simulink model "coremodel"  (R2026a)
settings: Solver=ode23t  StopTime=12  MaxStep=1e-4  RelTol=1e-4
values from neighbouring files (symbols this model uses):
  Bshaft = 2000    [init.m]    (also in isolator_config_demo.m)
  TorqueFullScaleNm = 10000    [init.m]    (also in isolator_config_demo.m)
  Ts = 0.001    [init.m]    (also in isolator_config_demo.m)
libraries: fl_lib x16, nesl_utility x10, ee_lib x1
settings Model: Creator=saranya  LastModifiedBy=saranya

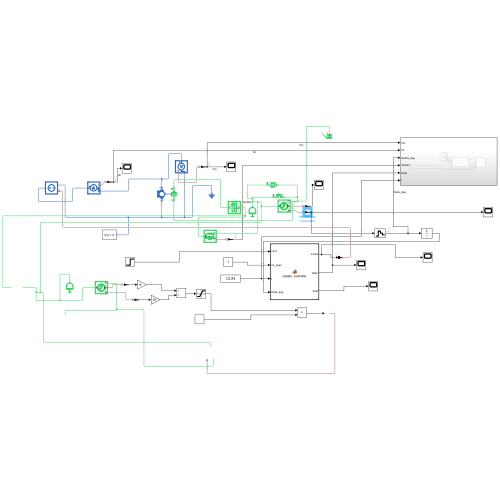
[thumbnail: Simulink's stored preview of the top-level diagram]
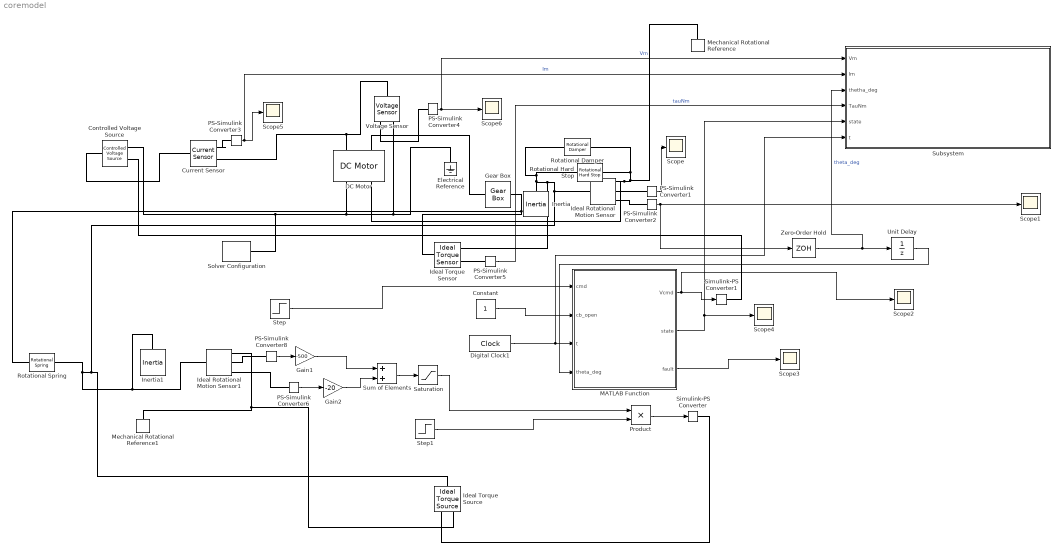
== system coremodel ==
  Constant : Constant
  Controlled Voltage Source : fl_lib/Electrical/Electrical Sources/Controlled Voltage Source
  Current Sensor : fl_lib/Electrical/Electrical Sensors/Current Sensor
  DC Motor : ee_lib/Electromechanical/Brushed Motors/DC Motor  field_option=ee.enum.field_option.pm  Rf=100 Ohm  Lf=1 H  Laf=0.15 H  If0=0 A  parameterization=ee.enum.dcparam_option.circuit_param  Ra=5 Ohm  La=0.05 H  emf_or_torque=ee.enum.emf_or_torque.ki  Kv=0.072e-3 V/rpm  Ki=0.5 N*m/A  T_stall=0.24e-3 N*m  w_max=19100 rpm  w_rated=15000 rpm  P_rated=0.08 W  V_rated=1.5 V  lam_param=ee.enum.lam_param.damping  i_noload=0 A  V_i_noload=1.5 V  J=0.002 cm^2*g  lam=0.001 N*m*s/rad  speed0=0 rpm  alpha=3.93e-3 1/K  Tmeas=25 degC  thermal_mass=100 J/K  initial_temperature=25 degC
  Digital Clock1 : DigitalClock
  Electrical Reference : fl_lib/Electrical/Electrical Elements/Electrical Reference
  Gain1 : Gain  Gain=-500
  Gain2 : Gain  Gain=-20
  Gear Box : fl_lib/Mechanical/Mechanisms/Gear Box  ratio=600  t_in_specify=off  t_in_priority=None  t_in=0 N*m  t_in_nominal_specify=off  t_in_nominal_value=1  t_in_nominal_unit=N*m  t_out_specify=off  t_out_priority=None  t_out=0 N*m  t_out_nominal_specify=off  t_out_nominal_value=1  t_out_nominal_unit=N*m
  Ideal Rotational Motion Sensor : fl_lib/Mechanical/Mechanical Sensors/Ideal Rotational Motion Sensor  reference=foundation.enum.MeasurementReference.difference  acceleration_port=false  velocity_port=true  position_port=true  wrap_angle=false  offset=0 rad
  Ideal Rotational Motion Sensor1 : fl_lib/Mechanical/Mechanical Sensors/Ideal Rotational Motion Sensor  reference=foundation.enum.MeasurementReference.difference  acceleration_port=false  velocity_port=true  position_port=true  wrap_angle=false  offset=0 rad
  Ideal Torque Sensor : fl_lib/Mechanical/Mechanical Sensors/Ideal Torque Sensor
  Ideal Torque Source : fl_lib/Mechanical/Mechanical Sources/Ideal Torque Source
  Inertia : fl_lib/Mechanical/Rotational Elements/Inertia  inertia=10 kg*m^2  num_ports=foundation.enum.numPorts2.one  w_specify=off  w_priority=High  w=0 rad/s  w_nominal_specify=off  w_nominal_value=1  w_nominal_unit=rad/s  t_specify=off  t_priority=None  t=0 N*m  t_nominal_specify=off  t_nominal_value=1  t_nominal_unit=N*m
  Inertia1 : fl_lib/Mechanical/Rotational Elements/Inertia  inertia=10 kg*m^2  num_ports=foundation.enum.numPorts2.one  w_specify=off  w_priority=High  w=0 rad/s  w_nominal_specify=off  w_nominal_value=1  w_nominal_unit=rad/s  t_specify=off  t_priority=None  t=0 N*m  t_nominal_specify=off  t_nominal_value=1  t_nominal_unit=N*m
  MATLAB Function : MATLAB Function  TreatAsAtomicUnit=on
  Mechanical Rotational Reference : fl_lib/Mechanical/Rotational Elements/Mechanical Rotational Reference
  Mechanical Rotational Reference1 : fl_lib/Mechanical/Rotational Elements/Mechanical Rotational Reference
  PS-Simulink Converter{1,3..4,6,8} (5 alike) : nesl_utility/PS-Simulink Converter  PhysicalDomain=network_engine_domain  SubClassName=ps_output  LeftPortType=input  RightPortType=output  PseudoPeriodic=off  Frequencies=[]  VectorFormat=inherit  Unit=inherit  AffineConversion=off
  PS-Simulink Converter2 : nesl_utility/PS-Simulink Converter  PhysicalDomain=network_engine_domain  SubClassName=ps_output  LeftPortType=input  RightPortType=output  PseudoPeriodic=off  Frequencies=[]  VectorFormat=inherit  Unit=deg  AffineConversion=off
  PS-Simulink Converter5 : nesl_utility/PS-Simulink Converter  PhysicalDomain=network_engine_domain  SubClassName=ps_output  LeftPortType=input  RightPortType=output  PseudoPeriodic=off  Frequencies=[]  VectorFormat=inherit  Unit=N*m  AffineConversion=off
  Product : Product
  Rotational Damper : fl_lib/Mechanical/Rotational Elements/Rotational Damper  D=Bshaft N*m*s/rad  w_specify=off  w_priority=None  w=0 rad/s  w_nominal_specify=off  w_nominal_value=1  w_nominal_unit=rad/s  t_specify=off  t_priority=None  t=0 N*m  t_nominal_specify=off  t_nominal_value=1  t_nominal_unit=N*m
  Rotational Hard Stop : fl_lib/Mechanical/Rotational Elements/Rotational Hard Stop  upper_bnd=pi/2 rad  lower_bnd=0 rad  model=simscape.enum.hardstop.smooth  stiff_up=1e6 N*m/rad  stiff_low=1e6 N*m/rad  D_up=0.01 N*m*s/rad  D_low=0.01 N*m*s/rad  transition=0.001 rad  coeff_rest=0.7  w_tol=0.1 rad/s  trq_tol=0.001 N*m  w_specify=off  w_priority=None  w=0 rad/s  w_nominal_specify=off  w_nominal_value=1  w_nominal_unit=rad/s  t_specify=off  t_priority=None  t=0 N*m  t_nominal_specify=off  t_nominal_value=1  t_nominal_unit=N*m  phi_specify=off  phi_priority=High  phi=0 rad  phi_nominal_specify=off  phi_nominal_value=1  phi_nominal_unit=rad  M_specify=off  M_priority=None  M=0
  Rotational Spring : fl_lib/Mechanical/Rotational Elements/Rotational Spring  spr_rate=10 N*m/rad  w_specify=off  w_priority=None  w=0 rad/s  w_nominal_specify=off  w_nominal_value=1  w_nominal_unit=rad/s  t_specify=off  t_priority=None  t=0 N*m  t_nominal_specify=off  t_nominal_value=1  t_nominal_unit=N*m  phi_specify=off  phi_priority=High  phi=0 rad  phi_nominal_specify=off  phi_nominal_value=1  phi_nominal_unit=rad
  Saturation : Saturate  UpperLimit=100  LowerLimit=-100
  Scope{,1..6} (7 alike) : Scope
      Scope2 settings: DataLoggingVariableName=ScopeData2
      Scope3 settings: DataLoggingVariableName=ScopeData3
      Scope4 settings: DataLoggingVariableName=ScopeData4
      Scope5 settings: DataLoggingVariableName=ScopeData5
      Scope6 settings: DataLoggingVariableName=ScopeData6
  Simulink-PS Converter : nesl_utility/Simulink-PS Converter  PhysicalDomain=network_engine_domain  SubClassName=ps_input  LeftPortType=input  RightPortType=output  PseudoPeriodic=off  Frequencies=[]  NoiseDistribution=none  NoiseParameters=[]  Unit=1  AffineConversion=off  FilteringAndDerivatives=provide  SimscapeFilterOrder=1  InputFilterTimeConstant=0.001  UdotUserProvided=0
  Simulink-PS Converter1 : nesl_utility/Simulink-PS Converter  PhysicalDomain=network_engine_domain  SubClassName=ps_input  LeftPortType=input  RightPortType=output  PseudoPeriodic=off  Frequencies=[]  NoiseDistribution=none  NoiseParameters=[]  Unit=1  AffineConversion=off  FilteringAndDerivatives=provide  SimscapeFilterOrder=1  InputFilterTimeConstant=0.001  UdotUserProvided=0
  Solver Configuration : nesl_utility/Solver Configuration  PhysicalDomain=network_engine_domain  SubClassName=solver  LeftPortType=input  RightPortType=generic  Tones=[]  Harmonics=[]  SimulateNoise=off  Profile=off  UseLocalSampling=off  EnableSwitchedLinearOptims=on  FrequencyDomain=off  UseCCode=off  RelTol=0.001  AbsTol=0.001  MinStep=1e-09  ToWorkspace=off  RevertToSquareIcSolve=off  NumHomotopyIterations=100  PhasorMode=off  PhasorModeNumHarmonics=1  ConsistencySolver=NEWTON_XTOL_AFTER_FTOL  CanonicalOrdering=CANONICAL  OptimizeIntermediates=OPTIMIZED  IndexReductionMethod=DerivativeReplacement  DoDC=off  ResidualTolerance=1e-09  ConsistencyTolSource=GLOBAL  ConsistencyAbsTol=0.001  ConsistencyRelTol=0.001  ConsistencyTolFactor=0.001  UseLocalSolver=off  LocalSolverChoice=NE_BACKWARD_EULER_ADVANCER  ResolveIndetEquations=on  FunctionEvalNumThread=1  LocalSolverSampleTime=0.001  DoFixedCost=off  MaxNonlinIter=3  MaxModeIter=2  ComputeImpulses=off  ImpulseIterations=2  LinearAlgebra=auto  LinearAlgebraNumThread=0  EquationFormulation=NE_TIME_EF  DelaysMemoryBudget=1024  AutomaticFiltering=on  FilteringTimeConstant=0.001  PartitionStorageMethod=AS_NEEDED  PartitionMemoryBudget=1024  PartitionMethod=ROBUST  MultibodyUseLocalSolver=off  MultibodyLocalSolverChoice=ODE1  MultibodyLocalSolverSampleTime=0.001
  Step : Step  SampleTime=0
  Step1 : Step  Time=2  InitialValue=1  FinalValue=0  SampleTime=0
  Subsystem : Subsystem
  Sum of Elements : Sum
  Unit Delay : UnitDelay  SampleTime=0.001
  Voltage Sensor : fl_lib/Electrical/Electrical Sensors/Voltage Sensor
  Zero-Order Hold : ZeroOrderHold  SampleTime=Ts
  wires:
  PS-Simulink Converter1/1 -> Scope/1
  PS-Simulink Converter2/1 -> Scope1/1, Zero-Order Hold/1
  Zero-Order Hold/1 -> Subsystem/3(thetha_deg), Unit Delay/1  "theta_deg"
  Digital Clock1/1 -> MATLAB Function/3(t), Subsystem/6(t)
  MATLAB Function/1(Vcmd) -> Simulink-PS Converter1/1, Scope2/1
  MATLAB Function/2(state) -> Subsystem/5(state), Scope4/1
  MATLAB Function/3(fault) -> Scope3/1
  PS-Simulink Converter3/1 -> Subsystem/2(Im), Scope5/1  "Im"
  PS-Simulink Converter4/1 -> Subsystem/1(Vm), Scope6/1  "Vm"
  PS-Simulink Converter5/1 -> Subsystem/4(TauNm)  "tauNm"
  PS-Simulink Converter8/1 -> Gain1/1
  PS-Simulink Converter6/1 -> Gain2/1
  Gain1/1 -> Sum of Elements/1
  Gain2/1 -> Sum of Elements/2
  Sum of Elements/1 -> Saturation/1
  Saturation/1 -> Product/1
  Product/1 -> Simulink-PS Converter/1
  Step1/1 -> Product/2
  Unit Delay/1 -> MATLAB Function/4(theta_deg)
  Constant/1 -> MATLAB Function/2(cb_open)
  Step/1 -> MATLAB Function/1(cmd)
  connections:
  Current Sensor/RConn2 -- Voltage Sensor/LConn1 -- DC Motor/LConn1
  Controlled Voltage Source/RConn2 -- Solver Configuration/RConn1 -- Voltage Sensor/RConn2 -- Electrical Reference/LConn1 -- DC Motor/RConn1
  Current Sensor/LConn1 -- Controlled Voltage Source/LConn1
  DC Motor/LConn2 -- Gear Box/LConn1
  Rotational Damper/LConn1 -- Rotational Spring/RConn1 -- Inertia1/LConn1 -- Ideal Rotational Motion Sensor1/LConn1 -- Ideal Torque Source/LConn1 -- Ideal Rotational Motion Sensor/LConn1 -- Ideal Torque Sensor/RConn1 -- Inertia/LConn1 -- Rotational Hard Stop/LConn1
  Rotational Damper/RConn1 -- Rotational Hard Stop/RConn1 -- Mechanical Rotational Reference/LConn1 -- Ideal Rotational Motion Sensor/RConn1 -- DC Motor/RConn2
  Ideal Rotational Motion Sensor/RConn2 -- PS-Simulink Converter1/LConn1
  Ideal Rotational Motion Sensor/RConn3 -- PS-Simulink Converter2/LConn1
  Simulink-PS Converter1/RConn1 -- Controlled Voltage Source/RConn1
  Current Sensor/RConn1 -- PS-Simulink Converter3/LConn1
  Voltage Sensor/RConn1 -- PS-Simulink Converter4/LConn1
  PS-Simulink Converter5/LConn1 -- Ideal Torque Sensor/RConn2
  Ideal Torque Sensor/LConn1 -- Rotational Spring/LConn1 -- Gear Box/RConn1
  Ideal Rotational Motion Sensor1/RConn1 -- Ideal Torque Source/RConn2 -- Mechanical Rotational Reference1/LConn1
  PS-Simulink Converter6/LConn1 -- Ideal Rotational Motion Sensor1/RConn3
  Ideal Rotational Motion Sensor1/RConn2 -- PS-Simulink Converter8/LConn1
  Ideal Torque Source/RConn1 -- Simulink-PS Converter/RConn1

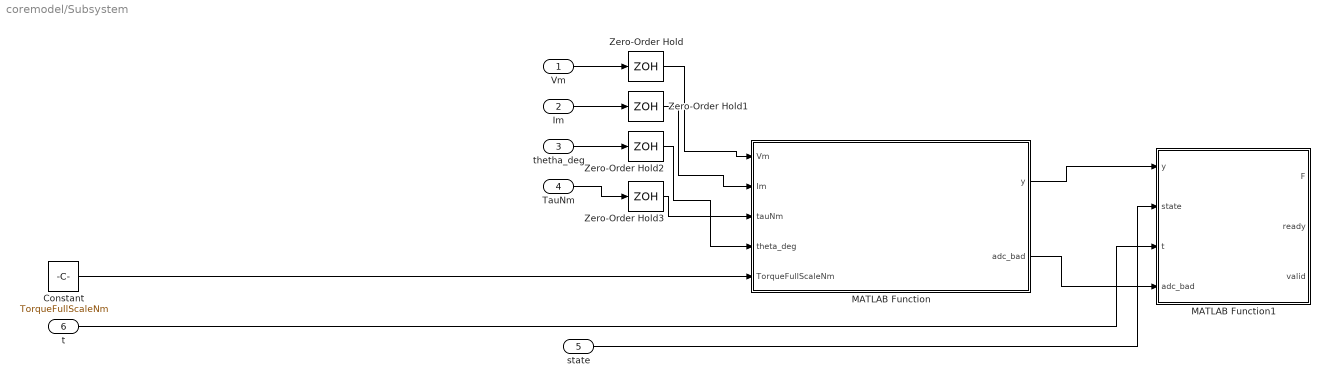
== system coremodel/Subsystem ==
  Vm : Inport
  Im : Inport  Port=2
  thetha_deg : Inport  Port=3
  TauNm : Inport  Port=4
  state : Inport  Port=5
  t : Inport  Port=6
  Constant : Constant  Value=TorqueFullScaleNm
  MATLAB Function : MATLAB Function  TreatAsAtomicUnit=on
  MATLAB Function1 : MATLAB Function  TreatAsAtomicUnit=on
  Zero-Order Hold{,1..3} (4 alike) : ZeroOrderHold  SampleTime=Ts
  wires:
  Im/1 -> Zero-Order Hold1/1
  Vm/1 -> Zero-Order Hold/1
  thetha_deg/1 -> Zero-Order Hold2/1
  Zero-Order Hold/1 -> MATLAB Function/1(Vm)
  Zero-Order Hold1/1 -> MATLAB Function/2(Im)
  Zero-Order Hold2/1 -> MATLAB Function/4(theta_deg)
  TauNm/1 -> Zero-Order Hold3/1
  MATLAB Function/2(adc_bad) -> MATLAB Function1/4(adc_bad)
  MATLAB Function/1(y) -> MATLAB Function1/1(y)
  state/1 -> MATLAB Function1/2(state)
  t/1 -> MATLAB Function1/3(t)
  Zero-Order Hold3/1 -> MATLAB Function/3(tauNm)
  Constant/1 -> MATLAB Function/5(TorqueFullScaleNm)

== matlab function coremodel/Subsystem/MATLAB Function ==
  data: Vm input; y output; Im input; tauNm input; theta_deg input; adc_bad output; TorqueFullScaleNm input
function [y, adc_bad] = mcxn547_adc_model(Vm, Im, tauNm, theta_deg, TorqueFullScaleNm)
%#codegen
% Paste ALL this code into the ADC MATLAB Function block.
% New fifth input: a Constant block with value TorqueFullScaleNm.
% y = [motor V, motor A, shaft torque N*m, output-shaft angle deg].
% Functional conditioning/quantization model, not MCXN547 emulation.
% The 16-bit / 3.3-V model is an illustrative configuration, not accuracy.

u = double([Vm, Im, tauNm, theta_deg]);
y = zeros(1,4);
adc_bad = ~all(isfinite(u)) || ~isfinite(TorqueFullScaleNm) || TorqueFullScaleNm <= 0;
if adc_bad
    return;
end

% EXAMPLE externally conditioned ranges, NOT a verified sensor circuit:
% Motor V: +/-150 V -> 0.15..3.15 V.
% Motor I: +/-25 A -> 0.15..3.15 V.
% Shaft torque: +/-TorqueFullScaleNm -> 0.15..3.15 V.
% Calibrated angle: 0..90 degrees -> 0.20..3.10 V.
v = [1.65 + 0.01*u(1), ...
    1.65 + 0.06*u(2), ...
    1.65 + 1.5*u(3)/TorqueFullScaleNm, ...
    0.20 + (2.90/90)*u(4)];
adc_bad = any(v <= 0) || any(v >= 3.3) || abs(tauNm) > TorqueFullScaleNm;
v = min(max(v,0),3.3);
counts = uint16(round(v*(65535/3.3)));
vq = double(counts)*(3.3/65535);
y = [(vq(1)-1.65)/0.01, ...
    (vq(2)-1.65)/0.06, ...
    (vq(3)-1.65)*TorqueFullScaleNm/1.5, ...
    (vq(4)-0.20)*(90/2.90)];
end

== matlab function coremodel/MATLAB Function ==
  settings: updateMethod=DISCRETE  sampleTime=0.001
  data: Vcmd output size=1; state output size=1; fault output size=1; cmd input size=1; cb_open input size=1; t input size=1; theta_deg input size=1
function [Vcmd,state,fault] = ...
    isolator_controller(cmd,cb_open,t,theta_deg)
%#codegen

% Requests:
% cmd =  1 : request closing
% cmd = -1 : request opening
% cmd =  0 : no new request
%
% States:
% 0 = OPEN
% 1 = CLOSING
% 2 = CLOSED
% 3 = OPENING
% 4 = FAULT
%
% Initial assumption: mechanism starts open at 0 degrees.



persistent s t_start

if isempty(s)
    s = 0;
    t_start = 0;
end

% Invalid angle measurement stops operation.
if ~isfinite(theta_deg)
    s = 4;
end

switch s
    case 0  % OPEN
        if cmd > 0.5 && cb_open > 0.5
            t_start = t;
            s = 1;
        end

    case 1  % CLOSING
        if cb_open <= 0.5
            s = 4;
        elseif theta_deg >= 89
            s = 2;
        elseif (t - t_start) >= 8
            s = 4;
        end

    case 2  % CLOSED
        if cmd < -0.5 && cb_open > 0.5
            t_start = t;
            s = 3;
        end

    case 3  % OPENING
        if cb_open <= 0.5
            s = 4;
        elseif theta_deg <= 1
            s = 0;
        elseif (t - t_start) >= 8
            s = 4;
        end

    otherwise  % FAULT remains latched
        s = 4;
end

% Generate the motor voltage command.
Vcmd = 0;

if s == 1
    Vcmd = 110;
elseif s == 3
    Vcmd = -110;
end

state = s;
fault = (s == 4);
end

== matlab function coremodel/Subsystem/MATLAB Function1 ==
  settings: updateMethod=DISCRETE  sampleTime=0.001
  data: y input; F output; state input; t input; adc_bad input; ready output; valid output


function [F,ready,valid] = operation_features(y,state,t,adc_bad)
%#codegen
%
% y(1) = motor voltage Vm [V]
% y(2) = motor current Im [A]
% y(3) = mechanism torque tau [N*m]
% y(4) = mechanism position theta [deg]
%
% F     = 18 x 1 feature vector
% ready = one-sample pulse when operation completes
% valid = measurement validity for the completed operation

%% ------------------------------------------------------------
% STATE DEFINITIONS
% Change if your controller uses different values
% -------------------------------------------------------------
STATE_OPEN    = 0;
STATE_CLOSING = 1;
STATE_CLOSED  = 2;
STATE_OPENING = 3;
STATE_FAULT   = 4;

%% ------------------------------------------------------------
% OUTPUTS
% -------------------------------------------------------------
F = zeros(18,1,'single');

ready = false;
valid = false;

%% ------------------------------------------------------------
% PERSISTENT VARIABLES
% -------------------------------------------------------------
persistent active
persistent badDuringOperation

persistent n

persistent tStart
persistent tPrevious

persistent thetaStart
persistent thetaFinal

persistent sumI2
persistent sumAbsI
persistent maxAbsI

persistent sumV
persistent minV
persistent maxV

persistent previousI
persistent previousV
persistent maxAbsDI
persistent maxAbsDV

persistent peakPower
persistent energyAbs

persistent sumAbsTau
persistent sumTau
persistent sumTau2
persistent peakAbsTau

persistent sumAbsOmega

persistent storedFeatures
persistent lastOperationValid

%% ------------------------------------------------------------
% INITIALIZATION
% -------------------------------------------------------------
if isempty(active)

    active = false;
    badDuringOperation = false;

    n = uint32(0);

    tStart = 0;
    tPrevious = 0;

    thetaStart = 0;
    thetaFinal = 0;

    sumI2 = 0;
    sumAbsI = 0;
    maxAbsI = 0;

    sumV = 0;
    minV = 0;
    maxV = 0;

    previousI = 0;
    previousV = 0;

    maxAbsDI = 0;
    maxAbsDV = 0;

    peakPower = 0;
    energyAbs = 0;

    sumAbsTau = 0;
    sumTau = 0;
    sumTau2 = 0;
    peakAbsTau = 0;

    sumAbsOmega = 0;

    storedFeatures = zeros(18,1,'single');

    lastOperationValid = false;
end

%% ------------------------------------------------------------
% INPUT EXTRACTION
% -------------------------------------------------------------
V = double(y(1));
I = double(y(2));
tau = double(y(3));
theta = double(y(4));

%% ------------------------------------------------------------
% DETERMINE WHETHER MECHANISM IS MOVING
% -------------------------------------------------------------
moving = ...
    (state == STATE_CLOSING) || ...
    (state == STATE_OPENING);

%% ------------------------------------------------------------
% START OF NEW OPERATION
% -------------------------------------------------------------
if moving && ~active

    active = true;

    badDuringOperation = logical(adc_bad);

    n = uint32(1);

    tStart = double(t);
    tPrevious = double(t);

    thetaStart = theta;
    thetaFinal = theta;

    sumI2 = I*I;
    sumAbsI = abs(I);
    maxAbsI = abs(I);

    sumV = V;
    minV = V;
    maxV = V;

    previousI = I;
    previousV = V;

    maxAbsDI = 0;
    maxAbsDV = 0;

    P = V*I;

    peakPower = abs(P);
    energyAbs = 0;

    sumAbsTau = abs(tau);
    sumTau = tau;
    sumTau2 = tau*tau;
    peakAbsTau = abs(tau);

    sumAbsOmega = 0;

%% ------------------------------------------------------------
% OPERATION IN PROGRESS
% -------------------------------------------------------------
elseif moving && active

    dt = double(t) - tPrevious;

    if dt > 0

        n = n + 1;

        %% Current
        sumI2 = sumI2 + I*I;
        sumAbsI = sumAbsI + abs(I);

        if abs(I) > maxAbsI
            maxAbsI = abs(I);
        end

        %% Voltage
        sumV = sumV + V;

        if V < minV
            minV = V;
        end

        if V > maxV
            maxV = V;
        end

        %% Current derivative
        dIdt = (I-previousI)/dt;

        if abs(dIdt) > maxAbsDI
            maxAbsDI = abs(dIdt);
        end

        %% Voltage derivative
        dVdt = (V-previousV)/dt;

        if abs(dVdt) > maxAbsDV
            maxAbsDV = abs(dVdt);
        end

        %% Electrical power
        P = V*I;

        if abs(P) > peakPower
            peakPower = abs(P);
        end

        %% Electrical energy consumed
        energyAbs = energyAbs + abs(P)*dt;

        %% Torque
        sumAbsTau = sumAbsTau + abs(tau);
        sumTau = sumTau + tau;
        sumTau2 = sumTau2 + tau*tau;

        if abs(tau) > peakAbsTau
            peakAbsTau = abs(tau);
        end

        %% Angular velocity
        omega = ...
            (theta-thetaFinal)/dt;

        sumAbsOmega = ...
            sumAbsOmega + abs(omega);

        %% Update previous sample
        previousI = I;
        previousV = V;

        thetaFinal = theta;

        tPrevious = double(t);

    end

    if adc_bad
        badDuringOperation = true;
    end

%% ------------------------------------------------------------
% END OF OPERATION
% -------------------------------------------------------------
elseif ~moving && active

    active = false;

    thetaFinal = theta;

    duration = double(t)-tStart;

    Nd = double(n);

    if Nd >= 2 && duration > 0

        %% Current
        I_rms = sqrt(sumI2/Nd);

        I_mean_abs = sumAbsI/Nd;

        %% Voltage
        V_mean = sumV/Nd;

        V_span = maxV-minV;

        %% Torque
        Tau_mean_abs = sumAbsTau/Nd;

        Tau_mean = sumTau/Nd;

        varianceTau = ...
            max(sumTau2/Nd - Tau_mean*Tau_mean,0);

        Tau_std = sqrt(varianceTau);

        %% Position
        travelAngle = ...
            abs(thetaFinal-thetaStart);

        %% Angular velocity
        Omega_mean_abs = ...
            sumAbsOmega/max(Nd-1,1);

        %% ----------------------------------------------------
        % FEATURE VECTOR
        % -----------------------------------------------------
        storedFeatures(1)  = single(I_rms);
        storedFeatures(2)  = single(maxAbsI);
        storedFeatures(3)  = single(I_mean_abs);

        storedFeatures(4)  = single(V_mean);
        storedFeatures(5)  = single(minV);
        storedFeatures(6)  = single(V_span);

        storedFeatures(7)  = single(maxAbsDI);
        storedFeatures(8)  = single(maxAbsDV);

        storedFeatures(9)  = single(peakPower);
        storedFeatures(10) = single(energyAbs);

        storedFeatures(11) = single(Tau_mean_abs);
        storedFeatures(12) = single(peakAbsTau);
        storedFeatures(13) = single(Tau_std);

        storedFeatures(14) = single(thetaStart);
        storedFeatures(15) = single(thetaFinal);

        storedFeatures(16) = single(travelAngle);
        storedFeatures(17) = single(duration);

        storedFeatures(18) = single(Omega_mean_abs);

        lastOperationValid = ...
            ~badDuringOperation;

        ready = true;
        valid = lastOperationValid;

    else

        lastOperationValid = false;

        ready = true;
        valid = false;

    end
end

%% ------------------------------------------------------------
% OUTPUT STORED VECTOR
% -------------------------------------------------------------
F = storedFeatures;

end
